simulink model "StateSpaceDerivation"  (R2018a)
settings: Solver=ode45  StartTime=0.0  StopTime=0.2  MaxStep=1e-4  RelTol=1e-3
undefined symbols (not defined in the file or in its folder): ssA, ssB, ssC
libraries: powerlib x24
settings Model: Creator=cmparedes  LastModifiedBy=erich

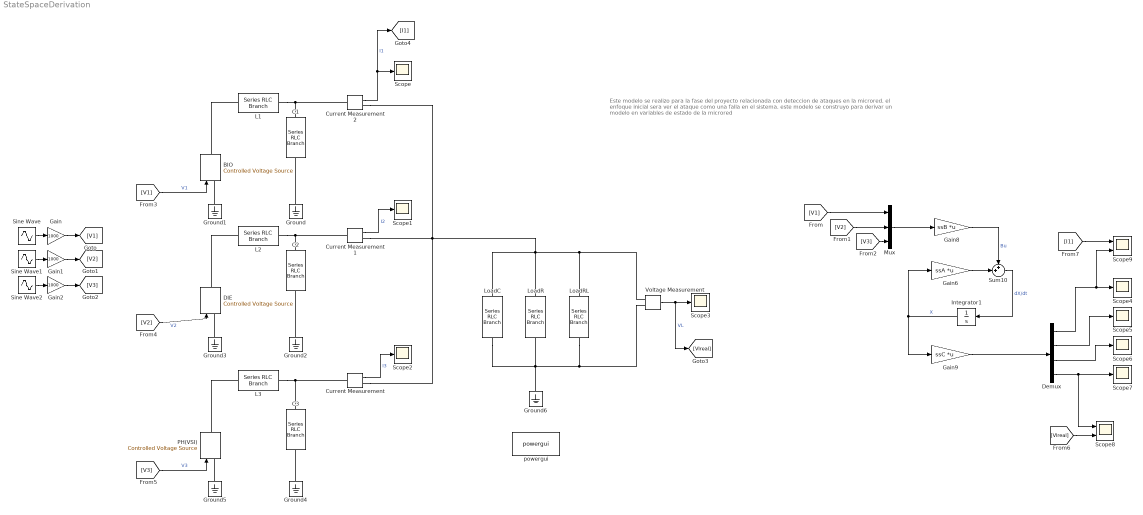
== system StateSpaceDerivation ==
  note: Este modelo se realizo para la fase del proyecto relacionada
      | con deteccion de ataques en la microred. el enfoque inicial
      | sera ver el ataque como una falla en el sistema.
      |
      | este modelo se construyo para derivar un modelo en variables
      | de estado de la microred
  BIO : powerlib/Electrical Sources/Controlled Voltage Source  Initialize=on  Source_Type=AC  Amplitude=0  Phase=0  Frequency=0  Measurements=None
  C1 : powerlib/Elements/Series RLC Branch  LConnTagsString=__new0  RConnTagsString=__new0  BranchType=C  Resistance=1  Inductance=1e-3  SetiL0=off  InitialCurrent=0  Capacitance=22e-6  Setx0=off  InitialVoltage=0  Measurements=None
  C2 : powerlib/Elements/Series RLC Branch  LConnTagsString=__new0  RConnTagsString=__new0  BranchType=C  Resistance=1  Inductance=1e-3  SetiL0=off  InitialCurrent=0  Capacitance=22e-6  Setx0=off  InitialVoltage=0  Measurements=None
  C3 : powerlib/Elements/Series RLC Branch  LConnTagsString=__new0  RConnTagsString=__new0  BranchType=C  Resistance=1  Inductance=1e-3  SetiL0=off  InitialCurrent=0  Capacitance=610e-6  Setx0=off  InitialVoltage=0  Measurements=None
  Current Measurement : powerlib/Measurements/Current Measurement  PhasorSimulation=off  OutputType=Complex  PSBequivalent=0
  Current Measurement1 : powerlib/Measurements/Current Measurement  PhasorSimulation=off  OutputType=Complex  PSBequivalent=0
  Current Measurement2 : powerlib/Measurements/Current Measurement  PhasorSimulation=off  OutputType=Complex  PSBequivalent=0
  DIE : powerlib/Electrical Sources/Controlled Voltage Source  Initialize=on  Source_Type=AC  Amplitude=0  Phase=0  Frequency=0  Measurements=None
  Demux : Demux
  Gain : Gain  Gain=1000
  Gain1 : Gain  Gain=1000
  Gain2 : Gain  Gain=1000
  Gain6 : Gain  Gain=ssA  Multiplication=Matrix(K*u)
  Gain8 : Gain  Gain=ssB  Multiplication=Matrix(K*u)
  Gain9 : Gain  Gain=ssC  Multiplication=Matrix(K*u)
  Ground{,1..6} (7 alike) : powerlib/Elements/Ground  LConnTagsString=a
  Integrator1 : Integrator
  L1 : powerlib/Elements/Series RLC Branch  LConnTagsString=__new0  RConnTagsString=__new0  BranchType=RL  Resistance=.1  Inductance=40e-3  SetiL0=off  InitialCurrent=0  Capacitance=1e-6  Setx0=off  InitialVoltage=0  Measurements=None
  L2 : powerlib/Elements/Series RLC Branch  LConnTagsString=__new0  RConnTagsString=__new0  BranchType=RL  Resistance=.1  Inductance=30e-3  SetiL0=off  InitialCurrent=0  Capacitance=1e-6  Setx0=off  InitialVoltage=0  Measurements=None
  L3 : powerlib/Elements/Series RLC Branch  LConnTagsString=__new0  RConnTagsString=__new0  BranchType=RL  Resistance=1e-3  Inductance=5e-3  SetiL0=off  InitialCurrent=0  Capacitance=1e-6  Setx0=off  InitialVoltage=0  Measurements=None
  LoadC : powerlib/Elements/Series RLC Branch  LConnTagsString=__new0  RConnTagsString=__new0  BranchType=C  Resistance=1  Inductance=1e-3  SetiL0=off  InitialCurrent=0  Capacitance=2000e-6  Setx0=off  InitialVoltage=0  Measurements=None
  LoadR : powerlib/Elements/Series RLC Branch  LConnTagsString=__new0  RConnTagsString=__new0  BranchType=R  Resistance=10  Inductance=1e-3  SetiL0=off  InitialCurrent=0  Capacitance=1e-6  Setx0=off  InitialVoltage=0  Measurements=None
  LoadRL : powerlib/Elements/Series RLC Branch  LConnTagsString=__new0  RConnTagsString=__new0  BranchType=RL  Resistance=10  Inductance=5.2  SetiL0=off  InitialCurrent=0  Capacitance=1e-6  Setx0=off  InitialVoltage=0  Measurements=None
  Mux : Mux  Inputs=3
  PH(VSI) : powerlib/Electrical Sources/Controlled Voltage Source  Initialize=on  Source_Type=AC  Amplitude=0  Phase=0  Frequency=0  Measurements=None
  Scope{,1..7} (8 alike) : Scope
  Scope8 : Scope  NumInputPorts=2
  Scope9 : Scope  NumInputPorts=2
  Sine Wave : Sin  Amplitude=.1  Frequency=60*2*pi  Phase=pi/2  SampleTime=0
  Sine Wave1 : Sin  Amplitude=.2  Frequency=60*2*pi  Phase=pi/4  SampleTime=0
  Sine Wave2 : Sin  Amplitude=.15  Frequency=60*2*pi  Phase=pi/8  SampleTime=0
  Sum10 : Sum  Inputs=++|
  Voltage Measurement : powerlib/Measurements/Voltage Measurement  PhasorSimulation=off  OutputType=Complex  PSBequivalent=0
  powergui : powerlib/powergui  Priority=1  SimulationMode=Continuous  SampleTime=50e-6  frequency=60  Iterations=50  frequencyindice=0  Pbase=100e6  ErrMax=1e-4  UnitsV=kV  UnitsW=MW  buscounter=0  FunctionMessages=off  echomessages=off  EnableUseOfTLC=off  CurrentSourceSwitches=off  DisableSnubberDevices=off  DisableRonSwitches=off  DisableVfSwitches=off  DisplayEquations=off  SolverType=Tustin/Backward Euler (TBE)  Interpol=off  ExternalGateDelay=off  methode=off  Ts=100  x0status=blocks  SPID=on  SwTol=0  HookPort=off  RestoreLinks=warning  ResistiveCurrentMeasurement=off  Frange=[0:2:500]  Ylog=off  Xlog=on  ShowGrid=off  save=off  variable=ZData  structure=0  ZoomFFT=off  StartTime=0.0  cycles=1  DisplayStyle=1  fundamental=60  FreqAxis=off  MaxFrequency=1000  frequencyindicesteady=1  RmsSteady=1  display=off
  wires:
  [V1] -> BIO/1  "V1"
  [V2] -> DIE/1  "V2"
  [V3] -> PH(VSI)/1  "V3"
  Current Measurement2/1 -> [I1], Scope/1  "I1"
  Current Measurement1/1 -> Scope1/1  "I2"
  Current Measurement/1 -> Scope2/1  "I3"
  Voltage Measurement/1 -> [Vlreal], Scope3/1  "VL"
  Integrator1/1 -> Gain9/1, Gain6/1  "X"
  Sum10/1 -> Integrator1/1  "dX/dt"
  Gain6/1 -> Sum10/2
  Gain8/1 -> Sum10/1  "Bu"
  Mux/1 -> Gain8/1
  [V1] -> Mux/1
  [V2] -> Mux/2
  [V3] -> Mux/3
  Sine Wave/1 -> Gain/1
  Sine Wave1/1 -> Gain1/1
  Sine Wave2/1 -> Gain2/1
  Gain9/1 -> Demux/1
  Demux/1 -> Scope9/2, Scope4/1
  Demux/2 -> Scope5/1
  Demux/3 -> Scope6/1
  Demux/4 -> Scope8/1, Scope7/1
  Gain/1 -> [V1]
  Gain1/1 -> [V2]
  Gain2/1 -> [V3]
  [Vlreal] -> Scope8/2
  [I1] -> Scope9/1
  connections:
  L1/LConn1 -- BIO/RConn1
  Ground/LConn1 -- C1/RConn1
  Ground1/LConn1 -- BIO/LConn1
  Ground2/LConn1 -- C2/RConn1
  Ground3/LConn1 -- DIE/LConn1
  L2/LConn1 -- DIE/RConn1
  L3/LConn1 -- PH(VSI)/RConn1
  Ground5/LConn1 -- PH(VSI)/LConn1
  Ground4/LConn1 -- C3/RConn1
  Ground6/LConn1 -- Voltage Measurement/LConn2 -- LoadRL/RConn1 -- LoadC/RConn1 -- LoadR/RConn1
  LoadC/LConn1 -- Current Measurement2/RConn1 -- Current Measurement/RConn1 -- Current Measurement1/RConn1 -- LoadR/LConn1 -- LoadRL/LConn1 -- Voltage Measurement/LConn1
  L3/RConn1 -- Current Measurement/LConn1 -- C3/LConn1
  L2/RConn1 -- Current Measurement1/LConn1 -- C2/LConn1
  L1/RConn1 -- Current Measurement2/LConn1 -- C1/LConn1
